simulink library "EEE481Arduino"  (R2016a)
settings: Solver=ode45  StartTime=0.0  StopTime=10.0  RelTol=1e-3
values from neighbouring files (symbols this model uses):
  Tsa = 1    [TempControlSysId.mat]
undefined symbols (not defined in the file or in its folder): dacNum, pinNum
libraries: simulink x7
settings Model: Creator=rsjoshi1  LastModifiedBy=rsjoshi1
settings DataIOCC: LimitDataPoints=on  SaveFormat=Array
settings DebuggingCC: SolverPrmCheckMsg=warning
settings HardwareCC: ProdBitPerPointer=32  ProdLargestAtomicFloat=None  ProdIntDivRoundTo=Undefined  ProdEndianess=Unspecified  ProdWordSize=32  ProdHWDeviceType=32-bit Generic
settings ModelReferenceCC: PropagateSignalLabelsOutOfModel=off
settings ConfigComp: CovSFcnEnable=off

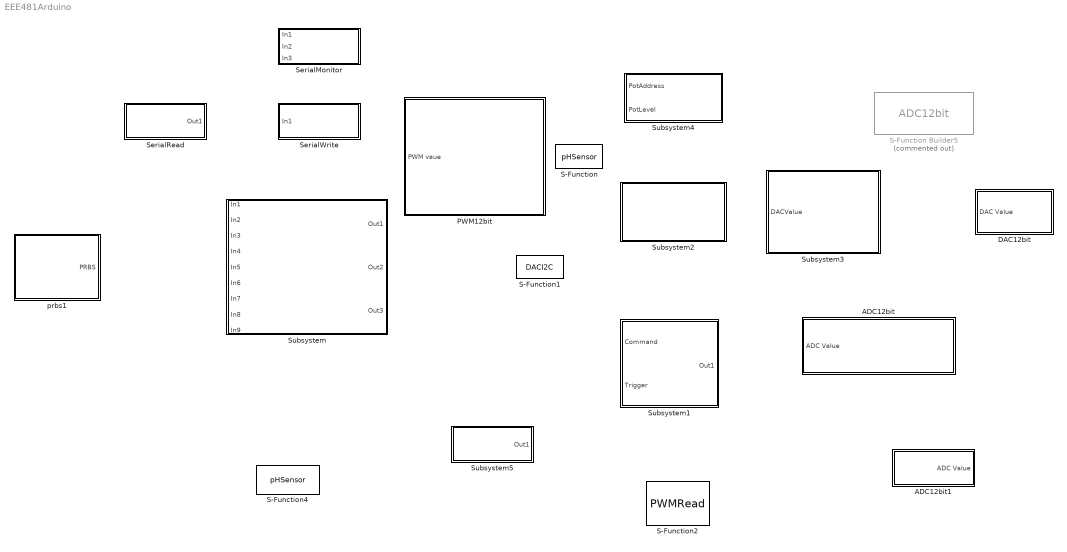
== system EEE481Arduino ==
  ADC12bit : Subsystem  mask{pinNum=5, Tsa=-1}
      mask prompts: pinNum "Analop Input Number"; Tsa "Sampling Time"
      mask Display: disp('12-Bit ADC')
  ADC12bit1 : Subsystem
  DAC12bit : Subsystem  mask{Tsa=-1, DACNum=1}
      mask prompts: Tsa "Sampling Time"; DACNum "DAC number(0 or 1)"
  PWM12bit : Subsystem  mask{PwmPort=8, Tsa=0}
      mask prompts: PwmPort "Pwm Port Number"; Tsa "Samping time"
      mask Display: disp('12-bit PWM write')
  S-Function : S-Function  FunctionName=pHSensor  Parameters=int8(0)  SFunctionModules=pHSensor_wrapper  SFunctionDeploymentMode=off  EnableBusSupport=off
  S-Function Builder5 : S-Function  Commented=on  InitFcn=try, set_param(gcb,'FunctionName','ADC12bit'), end  FunctionName=ADC12bit  Parameters=int8(pinNum)  SFunctionModules=ADC12bit_wrapper  SFunctionDeploymentMode=off  EnableBusSupport=off  mask(S-Function Builder){}
      mask help: Simulink:masks:SFunctionBuilder_MD
      mask init:
      | val = [[.9  0.75 0.75 1 1 .9 .9 1]',[1 1 0.75 0.75 .9 .9 1 .9]'];try , sys = get_param(gcb,'SfunBuilderFcnName');if isempty(sys), sys = get_param(gcb,'FunctionName'); end,catch, sys = get_param(gcb,'FunctionName'); end
      settings: CopyFcn=set_param(gcbh,'LinkStatus','none')  PreSaveFcn=try, set_param(gcb,'FunctionName','ADC12bit'), end  OpenFcn=sfunctionwizard(gcbh)
      mask Display: plot(val(:,1),val(:,2)),disp(sys), port_label('output',1,'output')
  S-Function1 : S-Function  FunctionName=DACI2C  SFunctionModules=DACI2C_wrapper  SFunctionDeploymentMode=off  EnableBusSupport=off
  S-Function2 : S-Function  FunctionName=PWMRead  SFunctionModules=PWMRead_wrapper  SFunctionDeploymentMode=off  EnableBusSupport=off
  S-Function4 : S-Function  FunctionName=pHSensor  Parameters=int8(2)  SFunctionModules=pHSensor_wrapper  SFunctionDeploymentMode=off  EnableBusSupport=off
  SerialMonitor : Subsystem  mask{Parameter1=0}
      mask Display: disp('Serial Monitor')
  SerialRead : Subsystem  mask{serialNum=2, Ts=0}
      mask prompts: serialNum "Serial Number"
      mask Display: disp('Serial read')
  SerialWrite : Subsystem  mask{serialNum=2, Tsa=0}
      mask prompts: serialNum "Serial Number"; Tsa "Sampling Time"
      mask Display: disp('Serial Write')
  Subsystem : Subsystem  mask{Tsa=0, rate=0, per=0}
      mask prompts: Tsa "Samping time"; rate "Input Rate"; per "Precision"
      mask help:
      | Serial Monitor block forms comma seperated string with the values of all 9 input signals for  specified prcision.
      | It sends comma seperated strinf to the serial port 0(USB cable) for the multiples of sampling time
      | It reads serial port for user inputs at a rate of  sampling time x input rate.
      mask Display: disp('Serial Monitor 9')
  Subsystem1 : Subsystem  mask{PortNum=2, Tsa=0}
      mask prompts: PortNum "Serial Port Number"; Tsa "Sampling Time"
      mask help:
      | Command value 0 corresponds to command "C,0"
      | Command value 1 corresponds to command "C,1"
      | Command value 2 corresponds to command "R"
      |
      | Trigger value of 1 makes this block transmit the command to the serial port
      mask Display: disp('pHRead')
  Subsystem2 : Subsystem
      mask help:
      | It sets Arduino Due as I2C salve with the address of 0x29
      | This block receives 12-bit data from the I2C bus  and sets output voltage of DAC0 of Arduino Due.
      mask Display: disp('I2C DAC Slave Model')
  Subsystem3 : Subsystem  mask{Tsa=0.01, SlaveAdd=41}
      mask prompts: Tsa "Samping Time"; SlaveAdd "Slave Address"
      mask help:
      | DACvalue whould be between 0-4095
      |
      | Formula for DAC voltage is given below
      |
      | DAC voltage= 0.6667* DAC Value+0.1667
      mask Display: disp('I2C DAC')
  Subsystem4 : Subsystem  mask{CS=53, Tsa=0}
      mask prompts: CS "SPI Address PIN"; Tsa "Sampling time"
      mask help:
      | This block is used to interface AD8402 digital potentiometer
      | Legal values of the potentiometer address are 0 and 1
      | Value whould be between 0-255
      mask Display: disp('SPI Potentiometer')
  Subsystem5 : Subsystem  mask{Tsa=0}
      mask prompts: Tsa "Sampling Time"
      mask help: This block reads PWM value of the signal on PWM 2 pin and outputs the values
      mask Display: disp('PWM Read')
  prbs1 : Subsystem  mask{Tsa=0, Tsw=0, Lz=0, Lv=0, Nc=0, initLevel=0}
      mask prompts: Tsa "Sample Time(s)"; Tsw "Time to switch(s)"; Lz "Leading Zeros(s)"; Lv "Switching Levels"; Nc "Number of Cycles"; initLevel "Initial level"
      mask Display: disp('PRBS generator')

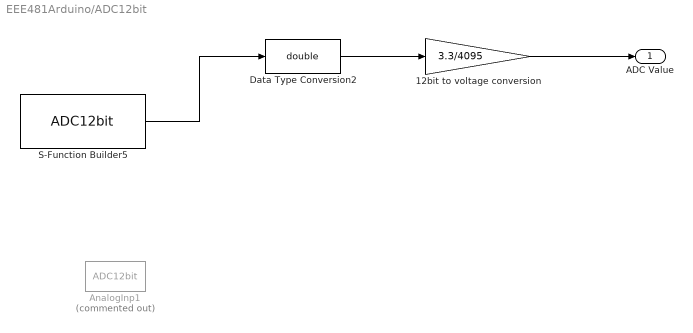
== system EEE481Arduino/ADC12bit ==
  12bit to voltage conversion : Gain  Gain=3.3/4095  SaturateOnIntegerOverflow=on  OutDataTypeStr=Inherit: Same as input  ParamDataTypeStr=Inherit: Same as input
  AnalogInp1 : S-Function  Commented=on  FunctionName=ADC12bit  Parameters=int8(pinNum)  SFunctionModules=ADC12bit_Wrapper  SFunctionDeploymentMode=off  EnableBusSupport=off
  Data Type Conversion2 : DataTypeConversion  OutDataTypeStr=double
  S-Function Builder5 : S-Function  InitFcn=try, set_param(gcb,'FunctionName','ADC12bit'), end  FunctionName=ADC12bit  Parameters=int8(pinNum)  SFunctionModules=ADC12bit_wrapper  SFunctionDeploymentMode=off  EnableBusSupport=off  mask(S-Function Builder){}
      mask help: Simulink:masks:SFunctionBuilder_MD
      mask init: same as EEE481Arduino/S-Function Builder5
      settings: CopyFcn=set_param(gcbh,'LinkStatus','none')  PreSaveFcn=try, set_param(gcb,'FunctionName','ADC12bit'), end  OpenFcn=sfunctionwizard(gcbh)
      mask Display: plot(val(:,1),val(:,2)),disp(sys), port_label('input',1,'u0'), port_label('output',1,'y0')
  ADC Value : Outport  SampleTime=Tsa
  wires:
  12bit to voltage conversion/1 -> ADC Value/1
  Data Type Conversion2/1 -> 12bit to voltage conversion/1
  S-Function Builder5/1 -> Data Type Conversion2/1

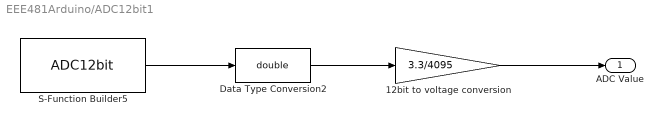
== system EEE481Arduino/ADC12bit1 ==
  12bit to voltage conversion : Gain  Gain=3.3/4095  SaturateOnIntegerOverflow=on  OutDataTypeStr=Inherit: Same as input  ParamDataTypeStr=Inherit: Same as input
  Data Type Conversion2 : DataTypeConversion  OutDataTypeStr=double
  S-Function Builder5 : S-Function  InitFcn=try, set_param(gcb,'FunctionName','ADC12bit'), end  FunctionName=ADC12bit  Parameters=int8(pinNum)  SFunctionModules=ADC12bit_wrapper  SFunctionDeploymentMode=off  EnableBusSupport=off  mask(S-Function Builder){}
      mask help: Simulink:masks:SFunctionBuilder_MD
      mask init: same as EEE481Arduino/S-Function Builder5
      settings: CopyFcn=set_param(gcbh,'LinkStatus','none')  PreSaveFcn=try, set_param(gcb,'FunctionName','ADC12bit'), end  OpenFcn=sfunctionwizard(gcbh)
      mask Display: plot(val(:,1),val(:,2)),disp(sys), port_label('output',1,'output')
  ADC Value : Outport  SampleTime=Tsa
  wires:
  12bit to voltage conversion/1 -> ADC Value/1
  Data Type Conversion2/1 -> 12bit to voltage conversion/1
  S-Function Builder5/1 -> Data Type Conversion2/1

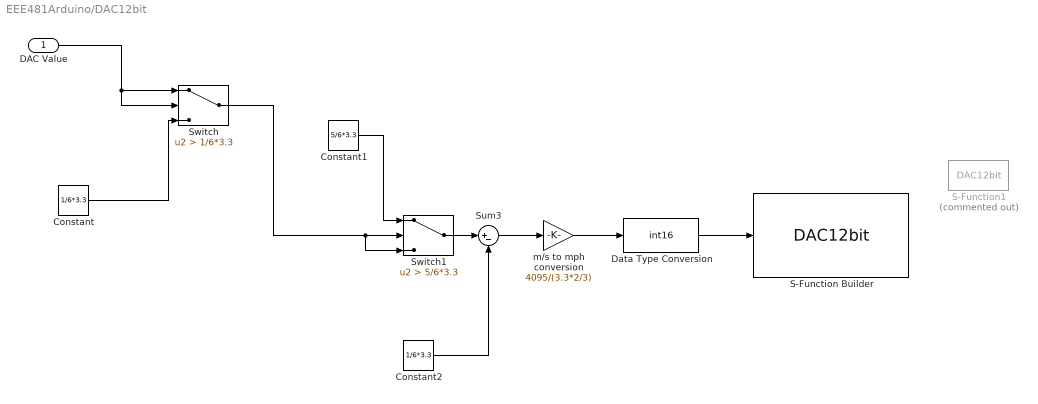
== system EEE481Arduino/DAC12bit ==
  DAC Value : Inport  SampleTime=Tsa
  Constant : Constant  Value=1/6*3.3
  Constant1 : Constant  Value=5/6*3.3
  Constant2 : Constant  Value=1/6*3.3
  Data Type Conversion : DataTypeConversion  OutDataTypeStr=int16
  S-Function Builder : S-Function  InitFcn=try, set_param(gcb,'FunctionName','DAC12bit'), end  FunctionName=DAC12bit  Parameters=int8(DACNum)  SFunctionModules=DAC12bit_wrapper  SFunctionDeploymentMode=off  EnableBusSupport=off  mask(S-Function Builder){}
      mask help: Simulink:masks:SFunctionBuilder_MD
      mask init: same as EEE481Arduino/S-Function Builder5
      settings: CopyFcn=set_param(gcbh,'LinkStatus','none')  PreSaveFcn=try, set_param(gcb,'FunctionName','DAC12bit'), end  OpenFcn=sfunctionwizard(gcbh)
      mask Display: plot(val(:,1),val(:,2)),disp(sys), port_label('input',1,'DACInput')
  S-Function1 : S-Function  Commented=on  FunctionName=DAC12bit  Parameters=int8(dacNum)  SFunctionModules=DAC12bit_wrapper  SFunctionDeploymentMode=off  EnableBusSupport=off
  Sum3 : Sum  Inputs=|+-
  Switch : Switch  Criteria=u2 > Threshold  Threshold=1/6*3.3
  Switch1 : Switch  Criteria=u2 > Threshold  Threshold=5/6*3.3
  m/s to mph conversion : Gain  Gain=4095/(3.3*2/3)  SaturateOnIntegerOverflow=on  OutDataTypeStr=Inherit: Same as input  ParamDataTypeStr=Inherit: Same as input
  wires:
  Constant2/1 -> Sum3/2
  Sum3/1 -> m/s to mph conversion/1
  Switch1/1 -> Sum3/1
  Constant1/1 -> Switch1/1
  Switch/1 -> Switch1/2, Switch1/3
  Constant/1 -> Switch/3
  DAC Value/1 -> Switch/1, Switch/2
  m/s to mph conversion/1 -> Data Type Conversion/1
  Data Type Conversion/1 -> S-Function Builder/1

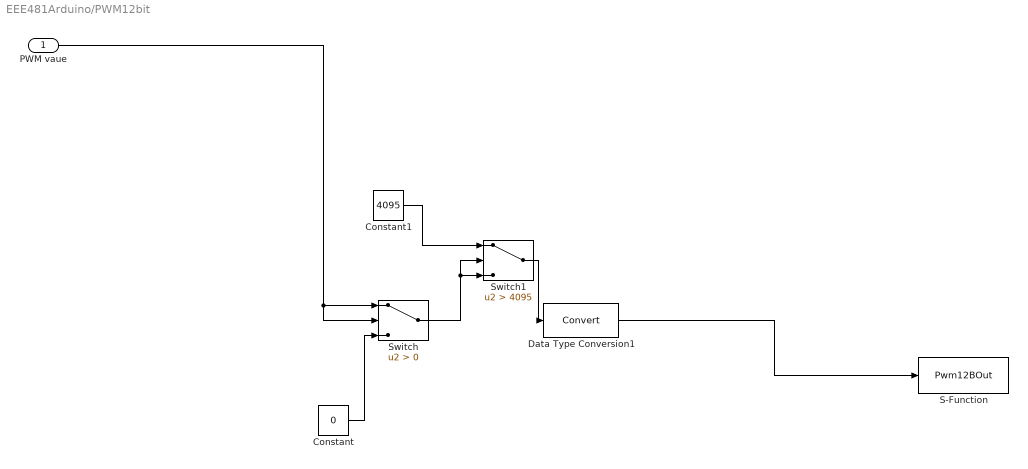
== system EEE481Arduino/PWM12bit ==
  PWM vaue : Inport  SampleTime=Tsa
  Constant : Constant  Value=0
  Constant1 : Constant  Value=4095
  Data Type Conversion1 : DataTypeConversion
  S-Function : S-Function  FunctionName=Pwm12BOut  Parameters=uint32(PwmPort)  SFunctionModules=Pwm12BOut_wrapper  SFunctionDeploymentMode=off  EnableBusSupport=off
  Switch : Switch  Criteria=u2 > Threshold
  Switch1 : Switch  Criteria=u2 > Threshold  Threshold=4095
  wires:
  PWM vaue/1 -> Switch/2, Switch/1
  Constant/1 -> Switch/3
  Switch/1 -> Switch1/2, Switch1/3
  Constant1/1 -> Switch1/1
  Switch1/1 -> Data Type Conversion1/1
  Data Type Conversion1/1 -> S-Function/1

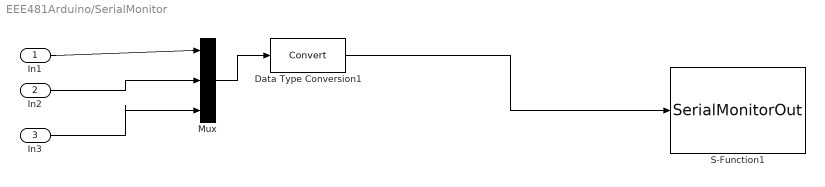
== system EEE481Arduino/SerialMonitor ==
  In1 : Inport
  In2 : Inport  Port=2
  In3 : Inport  Port=3
  Data Type Conversion1 : DataTypeConversion
  Mux : Mux  Inputs=3
  S-Function1 : S-Function  FunctionName=SerialMonitorOut  Parameters=int8(0)  SFunctionModules=SerialMonitorOut_wrapper  SFunctionDeploymentMode=off  EnableBusSupport=off
  wires:
  Data Type Conversion1/1 -> S-Function1/1
  In3/1 -> Mux/3
  In2/1 -> Mux/2
  In1/1 -> Mux/1
  Mux/1 -> Data Type Conversion1/1

== system EEE481Arduino/SerialRead ==
  Data Type Conversion4 : DataTypeConversion
  S-Function : S-Function  FunctionName=SerialIn  Parameters=int8(serialNum)  SFunctionModules=SerialIn_wrapper  SFunctionDeploymentMode=off  EnableBusSupport=off
  Out1 : Outport  SampleTime=Ts
  wires:
  Data Type Conversion4/1 -> Out1/1
  S-Function/1 -> Data Type Conversion4/1

== system EEE481Arduino/SerialWrite ==
  In1 : Inport  SampleTime=Tsa
  Data Type Conversion1 : DataTypeConversion
  S-Function : S-Function  FunctionName=SerialOut  Parameters=int8(serialNum)  SFunctionModules=SerialOut_wrapper  SFunctionDeploymentMode=off  EnableBusSupport=off
  wires:
  In1/1 -> Data Type Conversion1/1
  Data Type Conversion1/1 -> S-Function/1

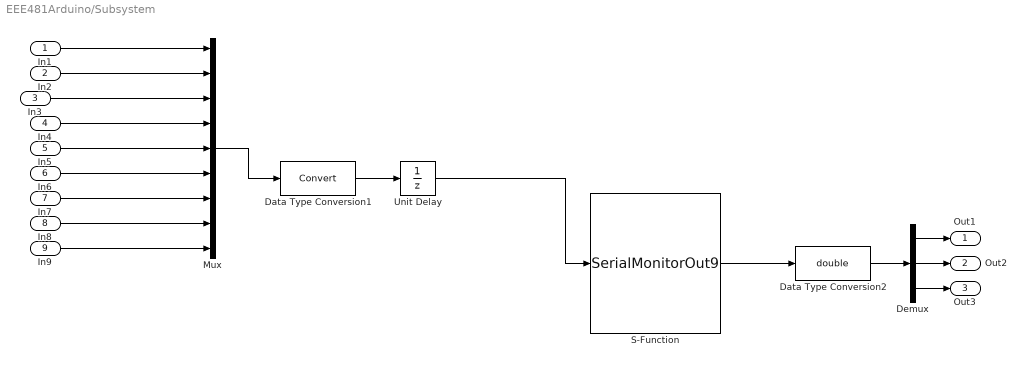
== system EEE481Arduino/Subsystem ==
  In1 : Inport  SampleTime=Tsa
  In2 : Inport  Port=2  SampleTime=Tsa
  In3 : Inport  Port=3  SampleTime=Tsa
  In4 : Inport  Port=4  SampleTime=Tsa
  In5 : Inport  Port=5  SampleTime=Tsa
  In6 : Inport  Port=6  SampleTime=Tsa
  In7 : Inport  Port=7  SampleTime=Tsa
  In8 : Inport  Port=8  SampleTime=Tsa
  In9 : Inport  Port=9  SampleTime=Tsa
  Data Type Conversion1 : DataTypeConversion
  Data Type Conversion2 : DataTypeConversion  OutDataTypeStr=double
  Demux : Demux  Outputs=3
  Mux : Mux  Inputs=9
  S-Function : S-Function  FunctionName=SerialMonitorOut9  Parameters=int8(0),int8(rate)  SFunctionModules=SerialMonitorOut9_wrapper  SFunctionDeploymentMode=off  EnableBusSupport=off
  Unit Delay : UnitDelay  SampleTime=Tsa
  Out1 : Outport  OutDataTypeStr=double  SampleTime=Tsa
  Out2 : Outport  Port=2  OutDataTypeStr=double  SampleTime=Tsa
  Out3 : Outport  Port=3  OutDataTypeStr=double  SampleTime=Tsa
  wires:
  Data Type Conversion1/1 -> Unit Delay/1
  In2/1 -> Mux/2
  In1/1 -> Mux/1
  Mux/1 -> Data Type Conversion1/1
  In6/1 -> Mux/6
  In5/1 -> Mux/5
  In4/1 -> Mux/4
  In9/1 -> Mux/9
  In8/1 -> Mux/8
  In7/1 -> Mux/7
  S-Function/1 -> Data Type Conversion2/1
  In3/1 -> Mux/3
  Data Type Conversion2/1 -> Demux/1
  Demux/1 -> Out1/1
  Demux/2 -> Out2/1
  Demux/3 -> Out3/1
  Unit Delay/1 -> S-Function/1

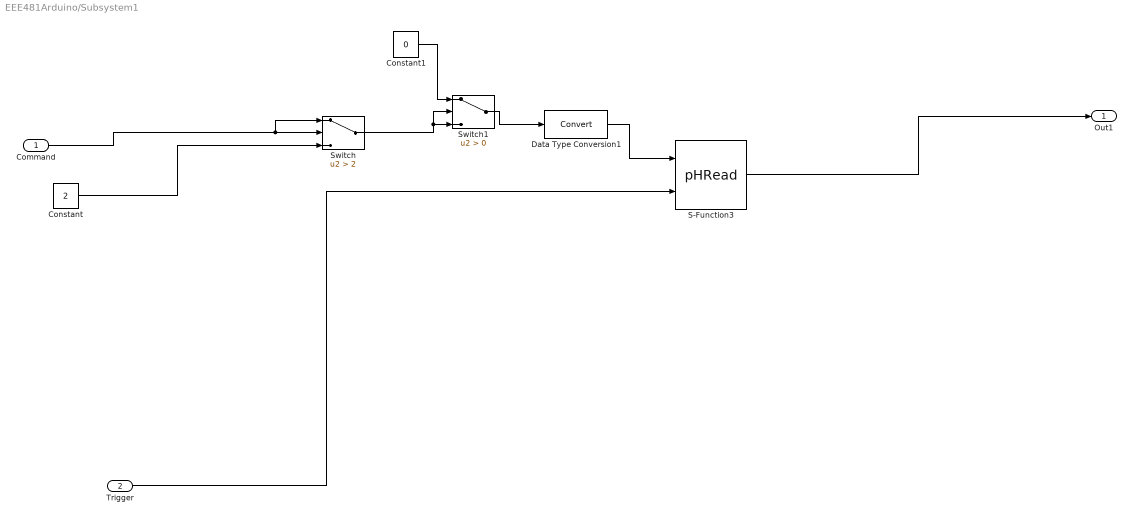
== system EEE481Arduino/Subsystem1 ==
  Command : Inport  SampleTime=Tsa
  Trigger : Inport  Port=2  SampleTime=Tsa
  Constant : Constant  Value=2
  Constant1 : Constant  Value=0
  Data Type Conversion1 : DataTypeConversion
  S-Function3 : S-Function  FunctionName=pHRead  Parameters=int8(PortNum)  SFunctionModules=pHRead_wrapper  SFunctionDeploymentMode=off  EnableBusSupport=off
      mask Display: disp('pHread')
  Switch : Switch  Criteria=u2 > Threshold  Threshold=2
  Switch1 : Switch  Criteria=u2 > Threshold
  Out1 : Outport
  wires:
  Trigger/1 -> S-Function3/2
  S-Function3/1 -> Out1/1
  Command/1 -> Switch/2, Switch/1
  Constant/1 -> Switch/3
  Switch/1 -> Switch1/2, Switch1/3
  Constant1/1 -> Switch1/1
  Switch1/1 -> Data Type Conversion1/1
  Data Type Conversion1/1 -> S-Function3/1

== system EEE481Arduino/Subsystem2 ==
  S-Function Builder12 : S-Function  InitFcn=try, set_param(gcb,'FunctionName','DACI2C1'), end  FunctionName=DACI2C1  SFunctionModules=DACI2C1_wrapper  SFunctionDeploymentMode=off  EnableBusSupport=off  mask(S-Function Builder){}
      mask help: Simulink:masks:SFunctionBuilder_MD
      mask init: same as EEE481Arduino/S-Function Builder5
      settings: CopyFcn=set_param(gcbh,'LinkStatus','none')  PreSaveFcn=try, set_param(gcb,'FunctionName','DACI2C1'), end  OpenFcn=sfunctionwizard(gcbh)
      mask Display:
      | plot(val(:,1),val(:,2))
      | disp(sys)

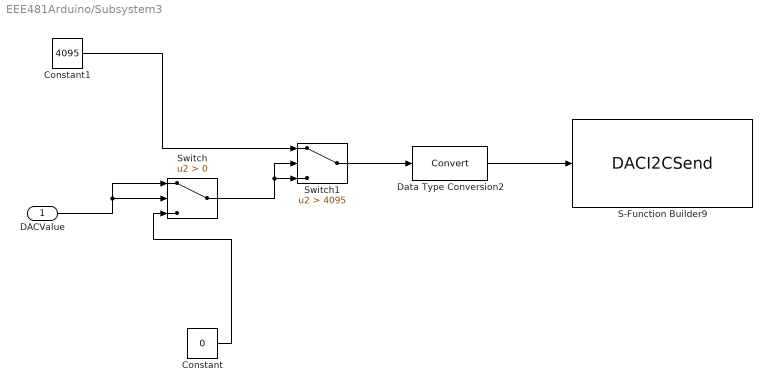
== system EEE481Arduino/Subsystem3 ==
  DACValue : Inport  SampleTime=Tsa
  Constant : Constant  Value=0
  Constant1 : Constant  Value=4095
  Data Type Conversion2 : DataTypeConversion
  S-Function Builder9 : S-Function  InitFcn=try, set_param(gcb,'FunctionName','DACI2CSend'), end  FunctionName=DACI2CSend  Parameters=int8(SlaveAdd)  SFunctionModules=DACI2CSend_wrapper  SFunctionDeploymentMode=off  EnableBusSupport=off  mask(S-Function Builder){}
      mask help: Simulink:masks:SFunctionBuilder_MD
      mask init: same as EEE481Arduino/S-Function Builder5
      settings: CopyFcn=set_param(gcbh,'LinkStatus','none')  PreSaveFcn=try, set_param(gcb,'FunctionName','DACI2CSend'), end  OpenFcn=sfunctionwizard(gcbh)
      mask Display: plot(val(:,1),val(:,2)),disp(sys), port_label('input',1,'DACValue')
  Switch : Switch  Criteria=u2 > Threshold
  Switch1 : Switch  Criteria=u2 > Threshold  Threshold=4095
  wires:
  DACValue/1 -> Switch/1, Switch/2
  Constant/1 -> Switch/3
  Switch/1 -> Switch1/2, Switch1/3
  Constant1/1 -> Switch1/1
  Switch1/1 -> Data Type Conversion2/1
  Data Type Conversion2/1 -> S-Function Builder9/1

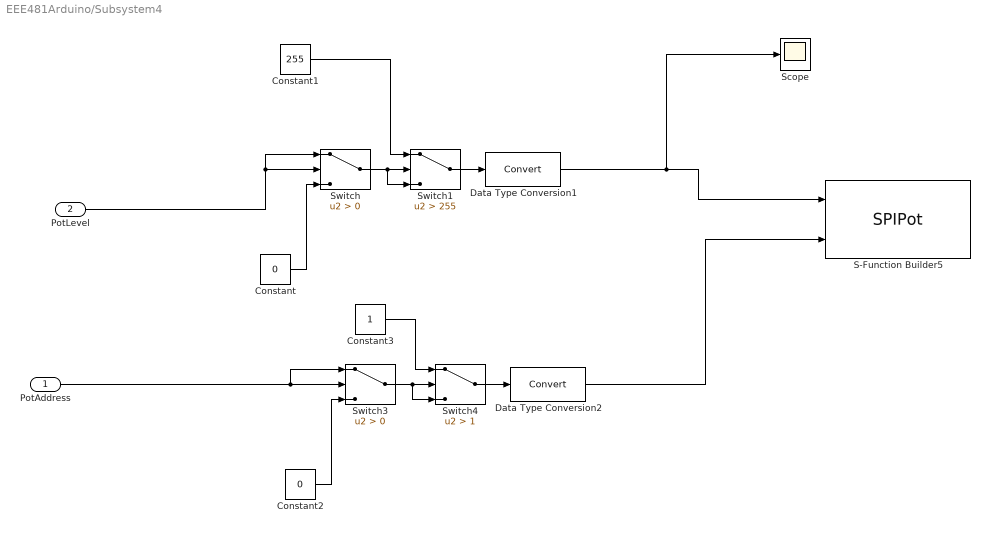
== system EEE481Arduino/Subsystem4 ==
  PotAddress : Inport  SampleTime=Tsa
  PotLevel : Inport  Port=2  SampleTime=Tsa
  Constant : Constant  Value=0
  Constant1 : Constant  Value=255
  Constant2 : Constant  Value=0
  Constant3 : Constant
  Data Type Conversion1 : DataTypeConversion
  Data Type Conversion2 : DataTypeConversion
  S-Function Builder5 : S-Function  InitFcn=try, set_param(gcb,'FunctionName','SPIPot'), end  FunctionName=SPIPot  Parameters=int8(CS)  SFunctionModules=SPIPot_wrapper  SFunctionDeploymentMode=off  EnableBusSupport=off  mask(S-Function Builder){}
      mask help: Simulink:masks:SFunctionBuilder_MD
      mask init: same as EEE481Arduino/S-Function Builder5
      settings: CopyFcn=set_param(gcbh,'LinkStatus','none')  PreSaveFcn=try, set_param(gcb,'FunctionName','SPIPot'), end  OpenFcn=sfunctionwizard(gcbh)
      mask Display: plot(val(:,1),val(:,2)),disp(sys), port_label('input',1,'PotLevel'), port_label('input',2,'PotAddress')
  Scope : Scope
  Switch : Switch  Criteria=u2 > Threshold
  Switch1 : Switch  Criteria=u2 > Threshold  Threshold=255
  Switch3 : Switch  Criteria=u2 > Threshold
  Switch4 : Switch  Criteria=u2 > Threshold  Threshold=1
  wires:
  PotLevel/1 -> Switch/2, Switch/1
  Constant/1 -> Switch/3
  Switch/1 -> Switch1/3, Switch1/2
  Constant1/1 -> Switch1/1
  Switch1/1 -> Data Type Conversion1/1
  Data Type Conversion1/1 -> Scope/1, S-Function Builder5/1
  PotAddress/1 -> Switch3/1, Switch3/2
  Constant2/1 -> Switch3/3
  Switch3/1 -> Switch4/2, Switch4/3
  Constant3/1 -> Switch4/1
  Switch4/1 -> Data Type Conversion2/1
  Data Type Conversion2/1 -> S-Function Builder5/2

== system EEE481Arduino/Subsystem5 ==
  Data Type Conversion2 : DataTypeConversion  OutDataTypeStr=double
  Gain : Gain  Gain=4095/1024
  S-Function2 : S-Function  FunctionName=PWMRead  SFunctionModules=PWMRead_wrapper  SFunctionDeploymentMode=off  EnableBusSupport=off
  Out1 : Outport  SampleTime=Tsa
  wires:
  S-Function2/1 -> Data Type Conversion2/1
  Data Type Conversion2/1 -> Gain/1
  Gain/1 -> Out1/1

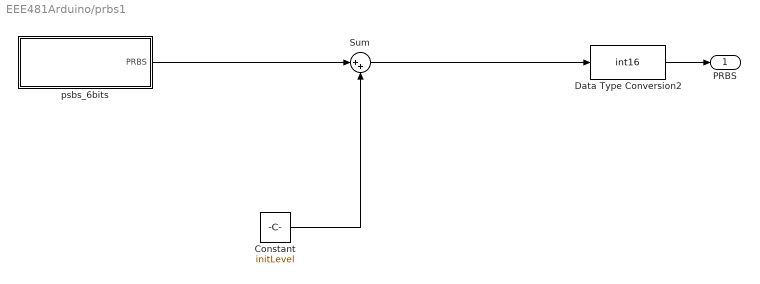
== system EEE481Arduino/prbs1 ==
  Constant : Constant  Value=initLevel
  Data Type Conversion2 : DataTypeConversion  OutDataTypeStr=int16
  Sum : Sum  Inputs=|++
  psbs_6bits : Subsystem  mask(PRBS with 8 shift registers){T=Tsa, Tsw=Tsw, Lz=Lz, Lv=Lv, Nc=Nc}
      mask prompts: T "Sample Time (s)"; Tsw "Time to switch (s)"; Lz "Leading Zeros (s)"; Lv "Switching Levels"; Nc "Number of Cycles"
      mask help:
      | Creates a PRBS signal using 6 shift registers.
      |     *Time to switch (Tsw) must be an integer multiple of Sample Time (T).
      |     *Leading zeros specify how long the PRBS will be zero, in seconds, before the levels begin shifting.
      |     *Level is the amplitude of the desired PRBS signal. Both + and - levels are equal
      |     *Number of cycles determines the number of full cycles generated. Each cycle is (2^6-1)*Tsw seconds long
  PRBS : Outport
  wires:
  Data Type Conversion2/1 -> PRBS/1
  psbs_6bits/1(PRBS) -> Sum/1
  Sum/1 -> Data Type Conversion2/1
  Constant/1 -> Sum/2

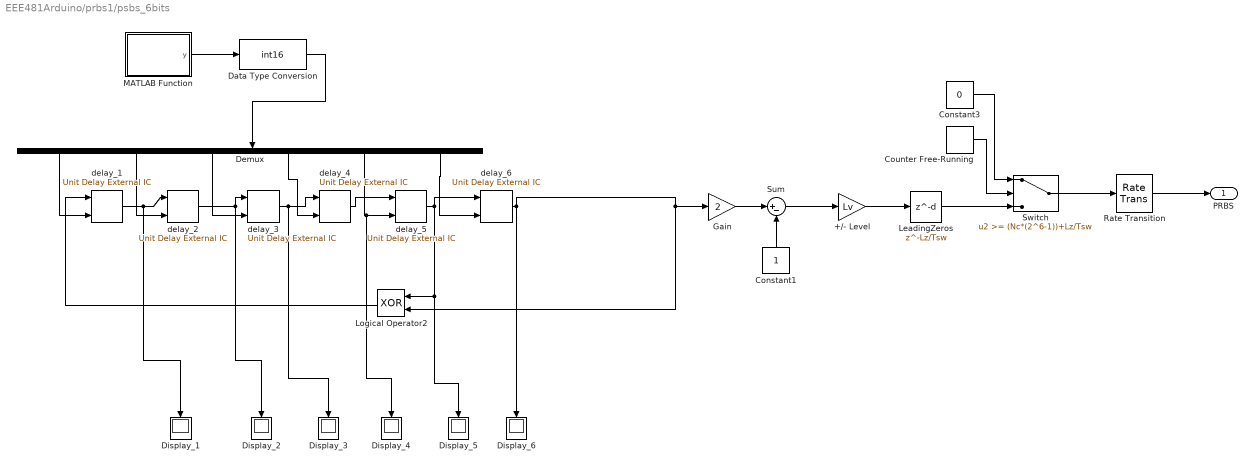
== system EEE481Arduino/prbs1/psbs_6bits ==
  +/- Level : Gain  Gain=Lv  SampleTime=Tsw
  Constant1 : Constant  SampleTime=Tsw
  Constant3 : Constant  Value=0  SampleTime=Tsw
  Counter Free-Running : simulink/Sources/Counter Free-Running  NumBits=32  tsamp=Tsw
  Data Type Conversion : DataTypeConversion  OutDataTypeStr=int16  SampleTime=Tsw
  Demux : Demux  Outputs=6
  Display_{1..6} (6 alike) : Display
  Gain : Gain  Gain=2  SampleTime=Tsw
  LeadingZeros : Delay  DelayLength=Lz/Tsw  InitialCondition=0  SampleTime=Tsw
  Logical Operator2 : Logic  Operator=XOR  AllPortsSameDT=off  OutDataTypeStr=fixdt(1,16)  SampleTime=Tsw
  MATLAB Function : MATLAB Function  TreatAsAtomicUnit=on
      settings: PermitHierarchicalResolution=ParametersOnly
  Rate Transition : RateTransition  OutPortSampleTime=T
  Sum : Sum  Inputs=|+-  SampleTime=Tsw
  Switch : Switch  Threshold=(Nc*(2^6-1))+Lz/Tsw  SampleTime=Tsw
  delay_{1..6} (6 alike) : simulink/Additional Math & Discrete/Additional Discrete/Unit Delay External IC  tsamp=Tsw
  PRBS : Outport
  wires:
  delay_5/1 -> Logical Operator2/1, Display_5/1, delay_6/1
  delay_2/1 -> Display_2/1, delay_3/1
  delay_3/1 -> Display_3/1, delay_4/1
  delay_4/1 -> delay_5/1
  delay_1/1 -> delay_2/1, Display_1/1
  delay_6/1 -> Logical Operator2/2, Gain/1, Display_6/1
  MATLAB Function/1(y) -> Data Type Conversion/1
  Demux/6 -> delay_6/2
  Demux/5 -> Display_4/1, delay_5/2
  Demux/4 -> delay_4/2
  Demux/3 -> delay_3/2
  Demux/2 -> delay_2/2
  Demux/1 -> delay_1/2
  Data Type Conversion/1 -> Demux/1
  Sum/1 -> +/- Level/1
  Gain/1 -> Sum/1
  Constant1/1 -> Sum/2
  Logical Operator2/1 -> delay_1/1
  Rate Transition/1 -> PRBS/1
  Counter Free-Running/1 -> Switch/2
  Switch/1 -> Rate Transition/1
  +/- Level/1 -> LeadingZeros/1
  Constant3/1 -> Switch/1
  LeadingZeros/1 -> Switch/3

== matlab function EEE481Arduino/prbs1/psbs_6bits/MATLAB Function ==
  data: y output
function y = fcn()
%#codegen
y = zeros(6,1);
% % s = de2bi(u,16);
% s = dec2bin(u,16);
s = ['1','1','0','1','0','0','1'];
y(1) = s(end-1)-48;
y(2) = s(end-2)-48;
y(3) = s(end-3)-48;
y(4) = s(end-4)-48;
y(5) = s(end-5)-48;
y(6) = s(end-6)-48;
